simulink model "q2_c_simulink_PD"  (R2013a)
settings: Solver=ode45  StartTime=0.0  StopTime=1.3  RelTol=1e-3
values from neighbouring files (symbols this model uses):
  Kd = Kd_temp    [f.m]
  Kp = Kp_temp    [f.m]
settings Model: Creator=obrien94  LastModifiedBy=obrien94

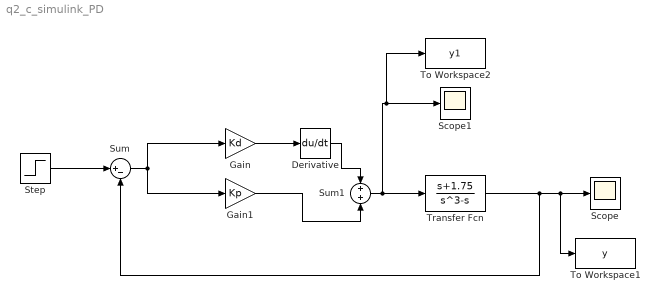
== system q2_c_simulink_PD ==
  Derivative : Derivative
  Gain : Gain  Gain=Kd
  Gain1 : Gain  Gain=Kp
  Scope : Scope
  Scope1 : Scope
  Step : Step  SampleTime=0
  Sum : Sum  Inputs=|+-
  Sum1 : Sum
  To Workspace1 : ToWorkspace  VariableName=y  SampleTime=-1  SaveFormat=Timeseries
  To Workspace2 : ToWorkspace  VariableName=y1  SampleTime=-1  SaveFormat=Timeseries
  Transfer Fcn : TransferFcn  Numerator=[1 1.75]  Denominator=[1 0 -1 0]
  wires:
  Step/1 -> Sum/1
  Gain/1 -> Derivative/1
  Derivative/1 -> Sum1/1
  Sum1/1 -> To Workspace2/1, Scope1/1, Transfer Fcn/1
  Gain1/1 -> Sum1/2
  Transfer Fcn/1 -> Sum/2, To Workspace1/1, Scope/1
  Sum/1 -> Gain/1, Gain1/1
